simulink library "lib_robotRP"  (Simulink 9.1)
settings: Solver=ode45  StartTime=0.0  StopTime=10.0  RelTol=1e-3
settings Model: SuppressorTable=22 serialization::archive 11 0 6 0 0 0 0 0  Creator=danes  LastModifiedBy=danes

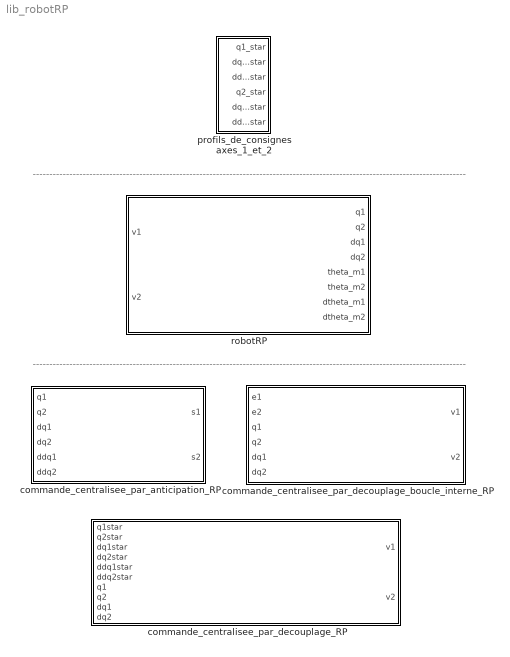
== system lib_robotRP ==
  note: ----------------------------------------------------------------------------------------------------------------------------------
  note: ----------------------------------------------------------------------------------------------------------------------------------
  commande_centralisee_par_anticipation_RP : Subsystem  mask(commande_feedforward_RP){}
      mask Display: fprintf('\ncompleter\nprealablement\nla S-function\nsf_loi_avant_RP\n');
  commande_centralisee_par_decouplage_RP : Subsystem  mask(commande_feedback_linearisant_RP){}
      mask Display: fprintf('\ncompleterprealablement la S-function\nsf_retour_linearisant_boucle_interne_RP\n\n(contient le rebouclage interne non lineaire)\n (et le rebouclage externe lineaire)\n');
  commande_centralisee_par_decouplage_boucle_interne_RP : Subsystem  mask(commande_feedback_linearisant_RP){}
      mask Display: fprintf('\ncompleter prealablement la S-function\nsf_retour_linearisant_boucle_interne_RP\n\n(a reboucler par un rebouclage externe !)\n');
  profils_de_consignes axes_1_et_2 : Subsystem  mask(profils_de_consignes_axes_1_et_2){}
  robotRP : Subsystem  mask(robotRP_commande_en_vitesse){vecteur_theta_dtheta_initial=[0 ; 100 ; 0 ; 0], m=15, gX=0, gY=-9.81, F1=0, F2=0, H1=0, H2=0, Km_sur_R=0.3, Jm=0.01, Beff=0.0125, r=1/200}
      mask prompts: vecteur_theta_dtheta_initial "Vecteur [theta_m1 ; theta_m2 ; dtheta_m1 ; dtheta_m2] à l'instant initial :"; m "Structure mécanique : Masse équivalente en O3"; gX "Structure mécanique : Champ de potentiel en O3 selon l'axe x"; gY "Structure mécanique : Champ de potentiel en O3 selon l'axe y"; F1 "Structure mécanique : Coefficient de frottement visqueux sur la liaison 1"; F2 "Structure mécanique : Coefficient de frottement visqueux sur la liaison 2"; H1 "Structure mécanique : Coefficient de frottement sec sur la liaison 1"; H2 "Structure mécanique : Coefficient de frottement sec sur la liaison 2"; Km_sur_R "Actionneurs : Km/R"; Jm "Actionneurs : Jm (cf. constante de temps = Jm/Beff)"; Beff "Actionneurs : Beff (cf. constante de temps = Jm/Beff)"; r "Rapport de réduction r (NE PAS OUBLIER DE MODIFIER LA CONDITION INITIALE EN CONSEQUENCE SI BESOIN)"
      mask Display: fprintf('ROBOT RP\n(avec actionneurs)\n(commandes en vitesse)');

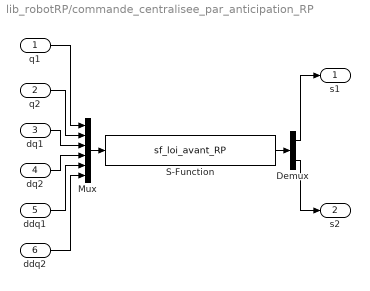
== system lib_robotRP/commande_centralisee_par_anticipation_RP ==
  q1 : Inport
  q2 : Inport  Port=2
  dq1 : Inport  Port=3
  dq2 : Inport  Port=4
  ddq1 : Inport  Port=5
  ddq2 : Inport  Port=6
  Demux : Demux  Outputs=2
  Mux : Mux  Inputs=6
  S-Function : S-Function  FunctionName=sf_loi_avant_RP  SFunctionDeploymentMode=off  EnableBusSupport=off
  s1 : Outport
  s2 : Outport  Port=2
  wires:
  q2/1 -> Mux/2
  q1/1 -> Mux/1
  dq1/1 -> Mux/3
  dq2/1 -> Mux/4
  Mux/1 -> S-Function/1
  ddq1/1 -> Mux/5
  ddq2/1 -> Mux/6
  Demux/2 -> s2/1
  Demux/1 -> s1/1
  S-Function/1 -> Demux/1

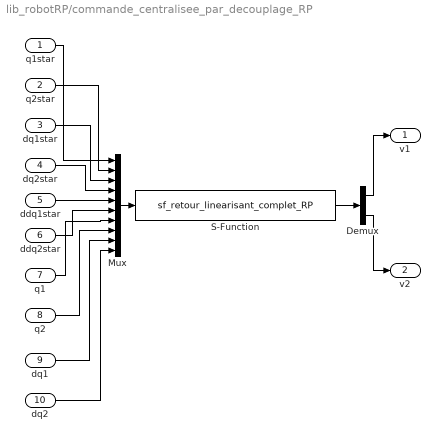
== system lib_robotRP/commande_centralisee_par_decouplage_RP ==
  q1star : Inport
  q2star : Inport  Port=2
  dq1star : Inport  Port=3
  dq2star : Inport  Port=4
  ddq1star : Inport  Port=5
  ddq2star : Inport  Port=6
  q1 : Inport  Port=7
  q2 : Inport  Port=8
  dq1 : Inport  Port=9
  dq2 : Inport  Port=10
  Demux : Demux  Outputs=2
  Mux : Mux  Inputs=10
  S-Function : S-Function  FunctionName=sf_retour_linearisant_complet_RP  SFunctionDeploymentMode=off  EnableBusSupport=off
  v1 : Outport
  v2 : Outport  Port=2
  wires:
  ddq2star/1 -> Mux/6
  ddq1star/1 -> Mux/5
  q2star/1 -> Mux/2
  q1star/1 -> Mux/1
  dq1star/1 -> Mux/3
  dq2star/1 -> Mux/4
  Mux/1 -> S-Function/1
  Demux/2 -> v2/1
  Demux/1 -> v1/1
  S-Function/1 -> Demux/1
  q1/1 -> Mux/7
  q2/1 -> Mux/8
  dq1/1 -> Mux/9
  dq2/1 -> Mux/10

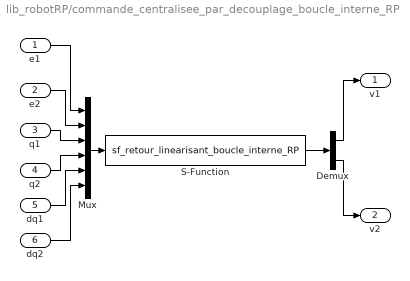
== system lib_robotRP/commande_centralisee_par_decouplage_boucle_interne_RP ==
  e1 : Inport
  e2 : Inport  Port=2
  q1 : Inport  Port=3
  q2 : Inport  Port=4
  dq1 : Inport  Port=5
  dq2 : Inport  Port=6
  Demux : Demux  Outputs=2
  Mux : Mux  Inputs=6
  S-Function : S-Function  FunctionName=sf_retour_linearisant_boucle_interne_RP  SFunctionDeploymentMode=off  EnableBusSupport=off
  v1 : Outport
  v2 : Outport  Port=2
  wires:
  S-Function/1 -> Demux/1
  Demux/1 -> v1/1
  Demux/2 -> v2/1
  Mux/1 -> S-Function/1
  q2/1 -> Mux/4
  q1/1 -> Mux/3
  e1/1 -> Mux/1
  e2/1 -> Mux/2
  dq1/1 -> Mux/5
  dq2/1 -> Mux/6

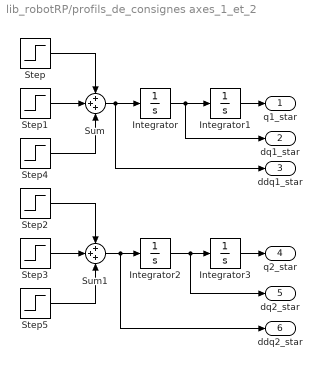
== system lib_robotRP/profils_de_consignes axes_1_et_2 ==
  Integrator : Integrator
  Integrator1 : Integrator
  Integrator2 : Integrator
  Integrator3 : Integrator  InitialCondition=0.5
  Step : Step  Before=pi/10  After=0  SampleTime=0
  Step1 : Step  Time=5  After=-pi/10  SampleTime=0
  Step2 : Step  Before=0.1  After=0  SampleTime=0
  Step3 : Step  Time=5  After=-0.1  SampleTime=0
  Step4 : Step  Time=6  After=pi/10  SampleTime=0
  Step5 : Step  Time=6  After=0.1  SampleTime=0
  Sum : Sum  Inputs=+++  SaturateOnIntegerOverflow=on  InputSameDT=on  OutDataTypeStr=Inherit: Same as first input
  Sum1 : Sum  Inputs=+++  SaturateOnIntegerOverflow=on  InputSameDT=on  OutDataTypeStr=Inherit: Same as first input
  q1_star : Outport
  dq1_star : Outport  Port=2
  ddq1_star : Outport  Port=3
  q2_star : Outport  Port=4
  dq2_star : Outport  Port=5
  ddq2_star : Outport  Port=6
  wires:
  Integrator3/1 -> q2_star/1
  Integrator1/1 -> q1_star/1
  Step5/1 -> Sum1/3
  Step4/1 -> Sum/3
  Step3/1 -> Sum1/2
  Step2/1 -> Sum1/1
  Step1/1 -> Sum/2
  Step/1 -> Sum/1
  Integrator/1 -> Integrator1/1, dq1_star/1
  Sum/1 -> Integrator/1, ddq1_star/1
  Integrator2/1 -> Integrator3/1, dq2_star/1
  Sum1/1 -> Integrator2/1, ddq2_star/1

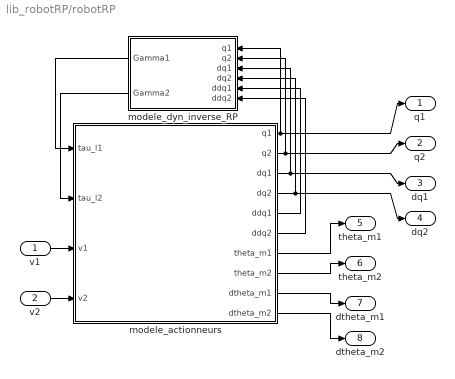
== system lib_robotRP/robotRP ==
  v1 : Inport
  v2 : Inport  Port=2
  modele_actionneurs : Subsystem  mask(modele_actionneurs){vecteur_theta_dtheta_initial=vecteur_theta_dtheta_initial, Km_sur_R=Km_sur_R, Jm=Jm, Beff=Beff, r=r}
      mask prompts: vecteur_theta_dtheta_initial "Vecteur [theta_m1 ; theta_m2 ; dtheta_m1 ; dtheta_m2] à l'instant initial :"; Km_sur_R "Km/R"; Jm "Jm (cf. constante de temps = Jm/Beff)"; Beff "Beff (cf. constante de temps = Jm/Beff)"; r "Rapport de réduction r"
      mask init:
      | theta_m1_initial = vecteur_theta_dtheta_initial(1);
      | theta_m2_initial = vecteur_theta_dtheta_initial(2);
      | dtheta_m1_initial = vecteur_theta_dtheta_initial(3);
      | dtheta_m2_initial = vecteur_theta_dtheta_initial(4);
  modele_dyn_inverse_RP : Subsystem  mask(modele_dyn_inverse_RP){m=m, gX=gX, gY=gY, F1=F1, F2=F2, H1=H1, H2=H2}
      mask prompts: m "Masse équivalente en O3"; gX "Champ de potentiel en O3 selon l'axe x"; gY "Champ de potentiel en O3 selon l'axe y"; F1 "Coefficient de frottement visqueux sur la liaison 1"; F2 "Coefficient de frottement visqueux sur la liaison 2"; H1 "Coefficient de frottement sec sur la liaison 1"; H2 "Coefficient de frottement sec sur la liaison 2"
  q1 : Outport
  q2 : Outport  Port=2
  dq1 : Outport  Port=3
  dq2 : Outport  Port=4
  theta_m1 : Outport  Port=5
  theta_m2 : Outport  Port=6
  dtheta_m1 : Outport  Port=7
  dtheta_m2 : Outport  Port=8
  wires:
  modele_actionneurs/4(dq2) -> dq2/1, modele_dyn_inverse_RP/4(dq2)
  modele_actionneurs/3(dq1) -> dq1/1, modele_dyn_inverse_RP/3(dq1)
  modele_actionneurs/2(q2) -> q2/1, modele_dyn_inverse_RP/2(q2)
  modele_actionneurs/1(q1) -> q1/1, modele_dyn_inverse_RP/1(q1)
  modele_actionneurs/10(dtheta_m2) -> dtheta_m2/1
  v2/1 -> modele_actionneurs/4(v2)
  modele_actionneurs/9(dtheta_m1) -> dtheta_m1/1
  modele_actionneurs/8(theta_m2) -> theta_m2/1
  modele_actionneurs/7(theta_m1) -> theta_m1/1
  v1/1 -> modele_actionneurs/3(v1)
  modele_actionneurs/6(ddq2) -> modele_dyn_inverse_RP/6(ddq2)
  modele_actionneurs/5(ddq1) -> modele_dyn_inverse_RP/5(ddq1)
  modele_dyn_inverse_RP/2(Gamma2) -> modele_actionneurs/2(tau_l2)
  modele_dyn_inverse_RP/1(Gamma1) -> modele_actionneurs/1(tau_l1)

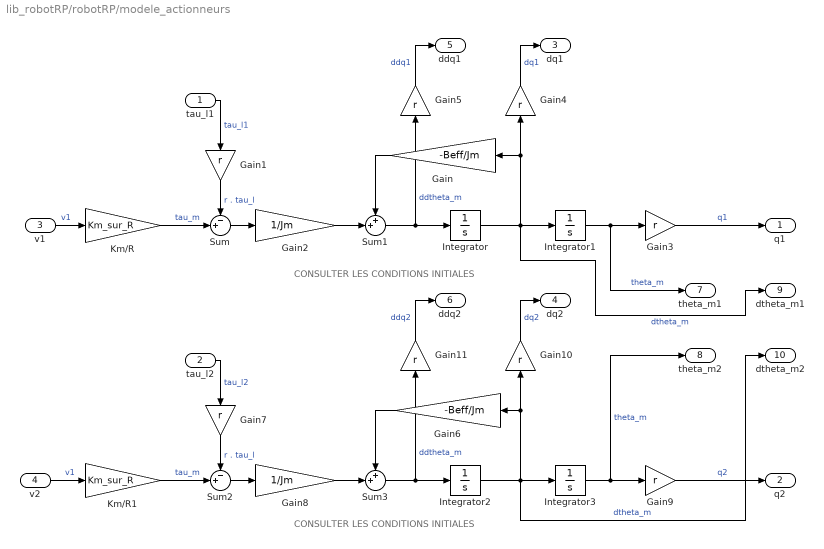
== system lib_robotRP/robotRP/modele_actionneurs ==
  note: CONSULTER LES CONDITIONS INITIALES
  note: CONSULTER LES CONDITIONS INITIALES
  tau_l1 : Inport
  tau_l2 : Inport  Port=2
  v1 : Inport  Port=3
  v2 : Inport  Port=4
  Gain : Gain  Gain=-Beff/Jm  SaturateOnIntegerOverflow=on  OutDataTypeStr=Inherit: Same as input  ParamDataTypeStr=Inherit: Same as input
  Gain{1,3..5,7,9..11} (8 alike) : Gain  Gain=r  SaturateOnIntegerOverflow=on  OutDataTypeStr=Inherit: Same as input  ParamDataTypeStr=Inherit: Same as input
  Gain2 : Gain  Gain=1/Jm  SaturateOnIntegerOverflow=on  OutDataTypeStr=Inherit: Same as input  ParamDataTypeStr=Inherit: Same as input
  Gain6 : Gain  Gain=-Beff/Jm  SaturateOnIntegerOverflow=on  OutDataTypeStr=Inherit: Same as input  ParamDataTypeStr=Inherit: Same as input
  Gain8 : Gain  Gain=1/Jm  SaturateOnIntegerOverflow=on  OutDataTypeStr=Inherit: Same as input  ParamDataTypeStr=Inherit: Same as input
  Integrator : Integrator  InitialCondition=dtheta_m1_initial
  Integrator1 : Integrator  InitialCondition=theta_m1_initial
  Integrator2 : Integrator  InitialCondition=dtheta_m2_initial
  Integrator3 : Integrator  InitialCondition=theta_m2_initial
  Km/R : Gain  Gain=Km_sur_R  SaturateOnIntegerOverflow=on  OutDataTypeStr=Inherit: Same as input  ParamDataTypeStr=Inherit: Same as input
  Km/R1 : Gain  Gain=Km_sur_R  SaturateOnIntegerOverflow=on  OutDataTypeStr=Inherit: Same as input  ParamDataTypeStr=Inherit: Same as input
  Sum : Sum  Inputs=-+|  SaturateOnIntegerOverflow=on  InputSameDT=on  OutDataTypeStr=Inherit: Same as first input
  Sum1 : Sum  Inputs=++|  SaturateOnIntegerOverflow=on  InputSameDT=on  OutDataTypeStr=Inherit: Same as first input
  Sum2 : Sum  Inputs=-+|  SaturateOnIntegerOverflow=on  InputSameDT=on  OutDataTypeStr=Inherit: Same as first input
  Sum3 : Sum  Inputs=++|  SaturateOnIntegerOverflow=on  InputSameDT=on  OutDataTypeStr=Inherit: Same as first input
  q1 : Outport
  q2 : Outport  Port=2
  dq1 : Outport  Port=3
  dq2 : Outport  Port=4
  ddq1 : Outport  Port=5
  ddq2 : Outport  Port=6
  theta_m1 : Outport  Port=7
  theta_m2 : Outport  Port=8
  dtheta_m1 : Outport  Port=9
  dtheta_m2 : Outport  Port=10
  wires:
  Gain2/1 -> Sum1/2
  Gain/1 -> Sum1/1
  Integrator/1 -> Integrator1/1, Gain/1, Gain4/1, dtheta_m1/1  "dtheta_m"
  Gain3/1 -> q1/1  "q1"
  Sum1/1 -> Integrator/1, Gain5/1  "ddtheta_m"
  Gain5/1 -> ddq1/1  "ddq1"
  Gain4/1 -> dq1/1  "dq1"
  Km/R/1 -> Sum/2  "tau_m"
  Gain1/1 -> Sum/1  "r . tau_l"
  v1/1 -> Km/R/1  "v1"
  Sum/1 -> Gain2/1
  Gain8/1 -> Sum3/2
  Gain6/1 -> Sum3/1
  Integrator2/1 -> Gain10/1, Gain6/1, Integrator3/1, dtheta_m2/1  "dtheta_m"
  Gain9/1 -> q2/1  "q2"
  Sum3/1 -> Gain11/1, Integrator2/1  "ddtheta_m"
  Gain11/1 -> ddq2/1  "ddq2"
  Gain10/1 -> dq2/1  "dq2"
  Km/R1/1 -> Sum2/2  "tau_m"
  Gain7/1 -> Sum2/1  "r . tau_l"
  v2/1 -> Km/R1/1  "v1"
  Sum2/1 -> Gain8/1
  tau_l2/1 -> Gain7/1  "tau_l2"
  tau_l1/1 -> Gain1/1  "tau_l1"
  Integrator1/1 -> Gain3/1, theta_m1/1  "theta_m"
  Integrator3/1 -> Gain9/1, theta_m2/1  "theta_m"

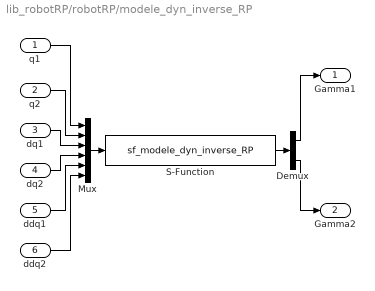
== system lib_robotRP/robotRP/modele_dyn_inverse_RP ==
  q1 : Inport
  q2 : Inport  Port=2
  dq1 : Inport  Port=3
  dq2 : Inport  Port=4
  ddq1 : Inport  Port=5
  ddq2 : Inport  Port=6
  Demux : Demux  Outputs=2
  Mux : Mux  Inputs=6
  S-Function : S-Function  FunctionName=sf_modele_dyn_inverse_RP  Parameters=m gX gY F1 F2 H1 H2  SFunctionDeploymentMode=off  EnableBusSupport=off
  Gamma1 : Outport
  Gamma2 : Outport  Port=2
  wires:
  S-Function/1 -> Demux/1
  Demux/1 -> Gamma1/1
  Demux/2 -> Gamma2/1
  ddq2/1 -> Mux/6
  ddq1/1 -> Mux/5
  Mux/1 -> S-Function/1
  dq2/1 -> Mux/4
  dq1/1 -> Mux/3
  q1/1 -> Mux/1
  q2/1 -> Mux/2
